simulink model "Appl_VentFault_CtrlModel"  (R2018b)
settings: configuration reference "CodeConfig_1_ms" (kept outside this file)
undefined symbols (not defined in the file): CAL_VentCmdOpenTime, CAL_VentCmdShortTime, FALSE, TRUE
libraries: DareLib x20, simulink x1
settings Model: Creator=Administrator  LastModifiedBy=Administrator
settings ConfigSetRef: SourceLocation=Base Workspace

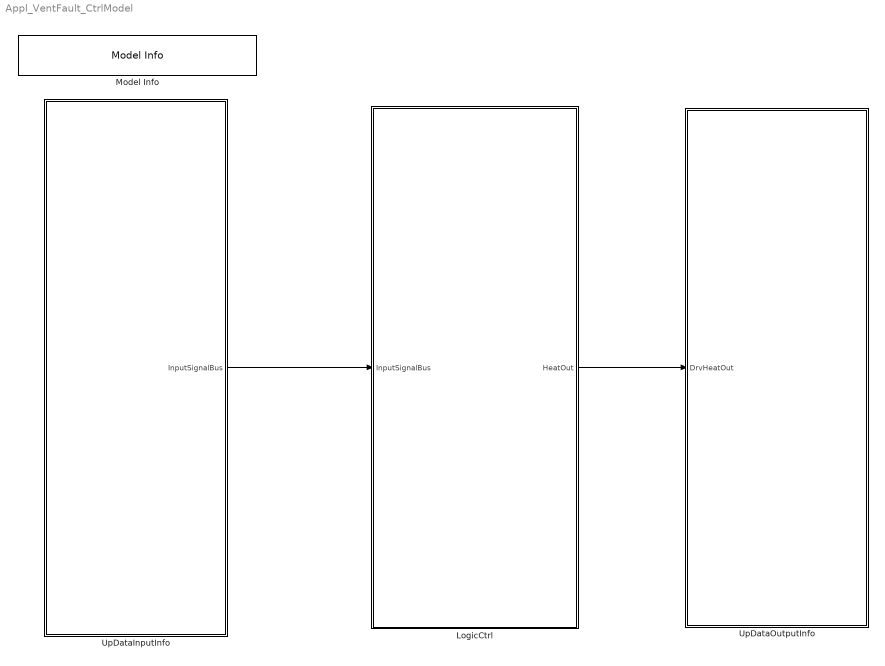
== system Appl_VentFault_CtrlModel ==
  LogicCtrl : Subsystem  Priority=2  TreatAsAtomicUnit=on
      settings: RTWSystemCode=Nonreusable function  RTWFcnNameOpts=Use subsystem name
  Model Info : simulink/Model-Wide Utilities/Model Info  Frame=on  DisplayStringWithTags=Version：%<ModelVersion>  HorizontalTextAlignment=Center  LeftAlignmentValue=0.5
  UpDataInputInfo : Subsystem  Priority=1  TreatAsAtomicUnit=on
      settings: RTWSystemCode=Nonreusable function  RTWFcnNameOpts=Use subsystem name
  UpDataOutputInfo : Subsystem  Priority=3  TreatAsAtomicUnit=on
      settings: RTWSystemCode=Nonreusable function  RTWFcnNameOpts=Use subsystem name
  wires:
  LogicCtrl/1(HeatOut) -> UpDataOutputInfo/1(DrvHeatOut)
  UpDataInputInfo/1(InputSignalBus) -> LogicCtrl/1(InputSignalBus)

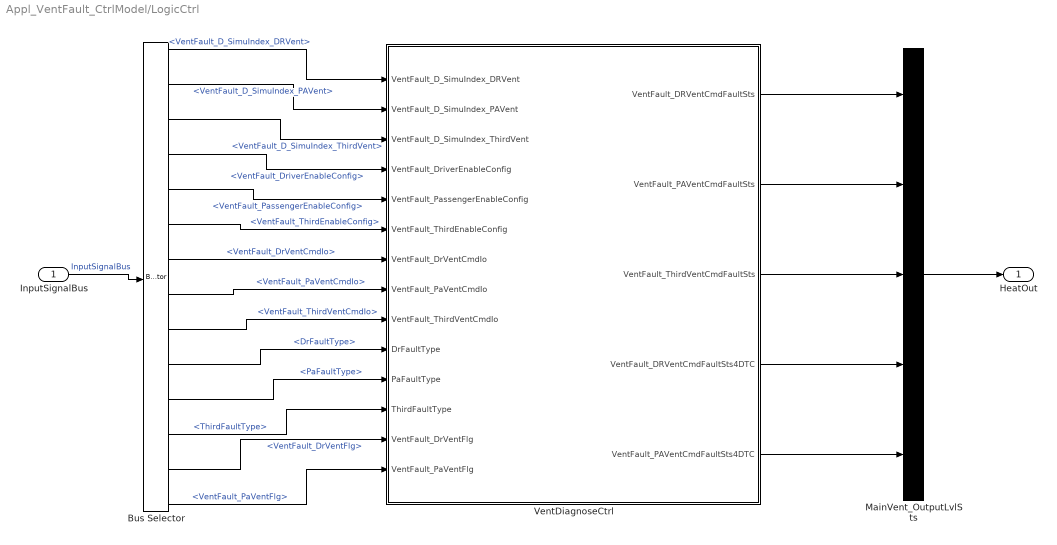
== system Appl_VentFault_CtrlModel/LogicCtrl ==
  InputSignalBus : Inport
  Bus Selector : BusSelector  OutputSignals=Rte_SignalBUs.VentFault_D_SimuIndex_DRVent,Rte_SignalBUs.VentFault_D_SimuIndex_PAVent,Rte_SignalBUs.VentFault_D_SimuIndex_ThirdVent,Rte_SignalBUs.VentFault_DriverEnableConfig,Rte_SignalBUs.VentFault_PassengerEnableConfig,Rte_SignalBUs.VentFault_ThirdEnableConfig,Rte_SignalBUs.VentFault_DrVentCmdIo,Rte_SignalBUs.VentFault_PaVentCmdIo,Rte_SignalBUs.VentFault_ThirdVentCmdIo,DrFaultType,PaFaultType,ThirdFaultType,Rte_SignalBUs.VentFault_DrVentFlg,Rte_SignalBUs.VentFault_PaVentFlg
  MainVent_OutputLvlSts : BusCreator  Inputs=5
  VentDiagnoseCtrl : Subsystem  Description=通风诊断逻辑处理
      settings: AttributesFormatString=%<Description>
  HeatOut : Outport
  wires:
  InputSignalBus/1 -> Bus Selector/1  "InputSignalBus"
  MainVent_OutputLvlSts/1 -> HeatOut/1
  Bus Selector/9 -> VentDiagnoseCtrl/9(VentFault_ThirdVentCmdIo)  "<VentFault_ThirdVentCmdIo>"
  Bus Selector/8 -> VentDiagnoseCtrl/8(VentFault_PaVentCmdIo)  "<VentFault_PaVentCmdIo>"
  Bus Selector/7 -> VentDiagnoseCtrl/7(VentFault_DrVentCmdIo)  "<VentFault_DrVentCmdIo>"
  Bus Selector/6 -> VentDiagnoseCtrl/6(VentFault_ThirdEnableConfig)  "<VentFault_ThirdEnableConfig>"
  Bus Selector/5 -> VentDiagnoseCtrl/5(VentFault_PassengerEnableConfig)  "<VentFault_PassengerEnableConfig>"
  Bus Selector/4 -> VentDiagnoseCtrl/4(VentFault_DriverEnableConfig)  "<VentFault_DriverEnableConfig>"
  Bus Selector/3 -> VentDiagnoseCtrl/3(VentFault_D_SimuIndex_ThirdVent)  "<VentFault_D_SimuIndex_ThirdVent>"
  Bus Selector/2 -> VentDiagnoseCtrl/2(VentFault_D_SimuIndex_PAVent)  "<VentFault_D_SimuIndex_PAVent>"
  Bus Selector/1 -> VentDiagnoseCtrl/1(VentFault_D_SimuIndex_DRVent)  "<VentFault_D_SimuIndex_DRVent>"
  VentDiagnoseCtrl/3(VentFault_ThirdVentCmdFaultSts) -> MainVent_OutputLvlSts/3
  VentDiagnoseCtrl/2(VentFault_PAVentCmdFaultSts) -> MainVent_OutputLvlSts/2
  VentDiagnoseCtrl/1(VentFault_DRVentCmdFaultSts) -> MainVent_OutputLvlSts/1
  VentDiagnoseCtrl/4(VentFault_DRVentCmdFaultSts4DTC) -> MainVent_OutputLvlSts/4
  VentDiagnoseCtrl/5(VentFault_PAVentCmdFaultSts4DTC) -> MainVent_OutputLvlSts/5
  Bus Selector/10 -> VentDiagnoseCtrl/10(DrFaultType)  "<DrFaultType>"
  Bus Selector/11 -> VentDiagnoseCtrl/11(PaFaultType)  "<PaFaultType>"
  Bus Selector/12 -> VentDiagnoseCtrl/12(ThirdFaultType)  "<ThirdFaultType>"
  Bus Selector/13 -> VentDiagnoseCtrl/13(VentFault_DrVentFlg)  "<VentFault_DrVentFlg>"
  Bus Selector/14 -> VentDiagnoseCtrl/14(VentFault_PaVentFlg)  "<VentFault_PaVentFlg>"

== system Appl_VentFault_CtrlModel/UpDataInputInfo ==
  InputSignalProcess : Subsystem  Description=数据处理
      settings: AttributesFormatString=%<Description>  RTWSystemCode=Nonreusable function  RTWFcnNameOpts=Use subsystem name
  RTE : Subsystem  Description=接口自动生成  TreatAsAtomicUnit=on
      settings: AttributesFormatString=%<Description>  RTWSystemCode=Nonreusable function  RTWFcnNameOpts=Use subsystem name
  InputSignalBus : Outport
  wires:
  RTE/1(RTE_Signal) -> InputSignalProcess/1(Rte_SignalBUs)
  InputSignalProcess/1(InputSignalBus) -> InputSignalBus/1

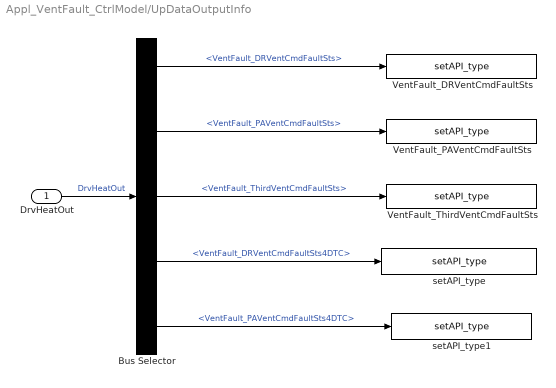
== system Appl_VentFault_CtrlModel/UpDataOutputInfo ==
  DrvHeatOut : Inport
  Bus Selector : BusSelector  OutputSignals=VentFault_DRVentCmdFaultSts,VentFault_PAVentCmdFaultSts,VentFault_ThirdVentCmdFaultSts,VentFault_DRVentCmdFaultSts4DTC,VentFault_PAVentCmdFaultSts4DTC
  VentFault_DRVentCmdFaultSts : DareLib/Dare/setAPI_type  g_funcname=Rte_SetVfb_DrVentCmdFaultSts  g_param=""  g_type=uint8  g_enum=enVentCmdFault  g_size=-1
      settings: AttributesFormatString=%<g_funcname>  SourceProductName=Dare Library
  VentFault_PAVentCmdFaultSts : DareLib/Dare/setAPI_type  g_funcname=Rte_SetVfb_PaVentCmdFaultSts  g_param=""  g_type=uint8  g_enum=enVentCmdFault  g_size=-1
      settings: AttributesFormatString=%<g_funcname>  SourceProductName=Dare Library
  VentFault_ThirdVentCmdFaultSts : DareLib/Dare/setAPI_type  g_funcname=Rte_SetVfb_ThirdVentCmdFaultSts  g_param=""  g_type=uint8  g_enum=enVentCmdFault  g_size=-1
      settings: AttributesFormatString=%<g_funcname>  SourceProductName=Dare Library
  setAPI_type : DareLib/Dare/setAPI_type  g_funcname=Rte_SetVfb_DrVentCmdFaultSts4DTC  g_param=""  g_type=uint8  g_size=-1
      settings: AttributesFormatString=%<g_funcname>  SourceProductName=Dare Library
  setAPI_type1 : DareLib/Dare/setAPI_type  g_funcname=Rte_SetVfb_PaVentCmdFaultSts4DTC  g_param=""  g_type=uint8  g_size=-1
      settings: AttributesFormatString=%<g_funcname>  SourceProductName=Dare Library
  wires:
  DrvHeatOut/1 -> Bus Selector/1  "DrvHeatOut"
  Bus Selector/2 -> VentFault_PAVentCmdFaultSts/1  "<VentFault_PAVentCmdFaultSts>"
  Bus Selector/1 -> VentFault_DRVentCmdFaultSts/1  "<VentFault_DRVentCmdFaultSts>"
  Bus Selector/3 -> VentFault_ThirdVentCmdFaultSts/1  "<VentFault_ThirdVentCmdFaultSts>"
  Bus Selector/4 -> setAPI_type/1  "<VentFault_DRVentCmdFaultSts4DTC>"
  Bus Selector/5 -> setAPI_type1/1  "<VentFault_PAVentCmdFaultSts4DTC>"

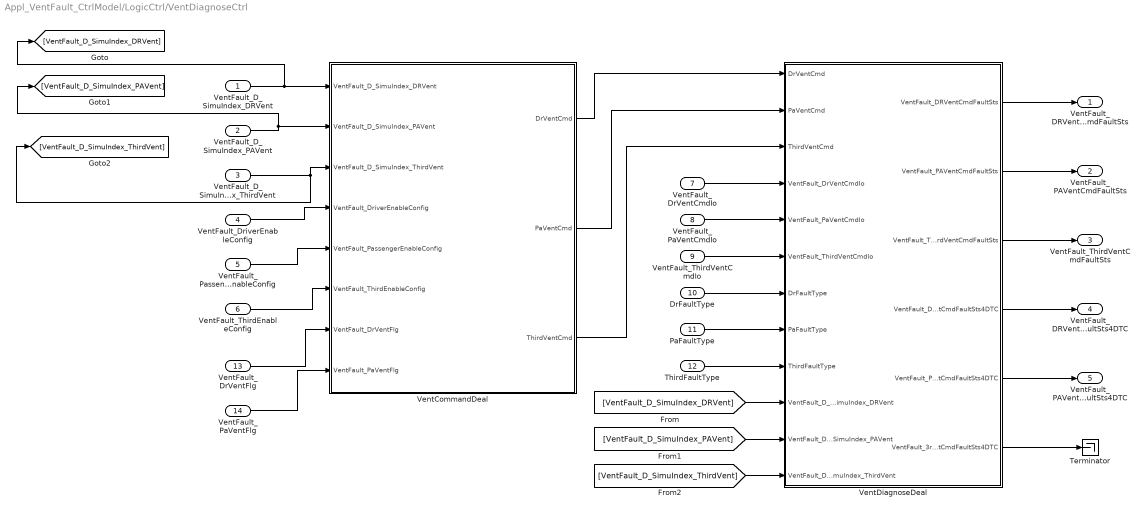
== system Appl_VentFault_CtrlModel/LogicCtrl/VentDiagnoseCtrl ==
  VentFault_D_SimuIndex_DRVent : Inport
  VentFault_D_SimuIndex_PAVent : Inport  Port=2
  VentFault_D_SimuIndex_ThirdVent : Inport  Port=3
  VentFault_DriverEnableConfig : Inport  Port=4
  VentFault_PassengerEnableConfig : Inport  Port=5
  VentFault_ThirdEnableConfig : Inport  Port=6
  VentFault_DrVentCmdIo : Inport  Port=7
  VentFault_PaVentCmdIo : Inport  Port=8
  VentFault_ThirdVentCmdIo : Inport  Port=9
  DrFaultType : Inport  Port=10
  PaFaultType : Inport  Port=11
  ThirdFaultType : Inport  Port=12
  VentFault_DrVentFlg : Inport  Port=13
  VentFault_PaVentFlg : Inport  Port=14
  Terminator : Terminator
  VentCommandDeal : Stateflow chart  TreatAsAtomicUnit=on
  VentDiagnoseDeal : Stateflow chart  TreatAsAtomicUnit=on
  VentFault_DRVentCmdFaultSts : Outport
  VentFault_PAVentCmdFaultSts : Outport  Port=2
  VentFault_ThirdVentCmdFaultSts : Outport  Port=3
  VentFault_DRVentCmdFaultSts4DTC : Outport  Port=4
  VentFault_PAVentCmdFaultSts4DTC : Outport  Port=5
  wires:
  VentDiagnoseDeal/3(VentFault_ThirdVentCmdFaultSts) -> VentFault_ThirdVentCmdFaultSts/1
  VentDiagnoseDeal/2(VentFault_PAVentCmdFaultSts) -> VentFault_PAVentCmdFaultSts/1
  VentDiagnoseDeal/1(VentFault_DRVentCmdFaultSts) -> VentFault_DRVentCmdFaultSts/1
  VentFault_D_SimuIndex_DRVent/1 -> [VentFault_D_SimuIndex_DRVent], VentCommandDeal/1(VentFault_D_SimuIndex_DRVent)
  VentFault_D_SimuIndex_PAVent/1 -> [VentFault_D_SimuIndex_PAVent], VentCommandDeal/2(VentFault_D_SimuIndex_PAVent)
  VentFault_D_SimuIndex_ThirdVent/1 -> [VentFault_D_SimuIndex_ThirdVent], VentCommandDeal/3(VentFault_D_SimuIndex_ThirdVent)
  VentCommandDeal/1(DrVentCmd) -> VentDiagnoseDeal/1(DrVentCmd)
  VentCommandDeal/2(PaVentCmd) -> VentDiagnoseDeal/2(PaVentCmd)
  VentCommandDeal/3(ThirdVentCmd) -> VentDiagnoseDeal/3(ThirdVentCmd)
  VentFault_DriverEnableConfig/1 -> VentCommandDeal/4(VentFault_DriverEnableConfig)
  VentFault_PassengerEnableConfig/1 -> VentCommandDeal/5(VentFault_PassengerEnableConfig)
  VentFault_ThirdEnableConfig/1 -> VentCommandDeal/6(VentFault_ThirdEnableConfig)
  VentFault_DrVentCmdIo/1 -> VentDiagnoseDeal/4(VentFault_DrVentCmdIo)
  VentFault_PaVentCmdIo/1 -> VentDiagnoseDeal/5(VentFault_PaVentCmdIo)
  VentFault_ThirdVentCmdIo/1 -> VentDiagnoseDeal/6(VentFault_ThirdVentCmdIo)
  VentDiagnoseDeal/5(VentFault_PAVentCmdFaultSts4DTC) -> VentFault_PAVentCmdFaultSts4DTC/1
  VentDiagnoseDeal/4(VentFault_DRVentCmdFaultSts4DTC) -> VentFault_DRVentCmdFaultSts4DTC/1
  DrFaultType/1 -> VentDiagnoseDeal/7(DrFaultType)
  PaFaultType/1 -> VentDiagnoseDeal/8(PaFaultType)
  ThirdFaultType/1 -> VentDiagnoseDeal/9(ThirdFaultType)
  VentDiagnoseDeal/6(VentFault_3rdVentCmdFaultSts4DTC) -> Terminator/1
  [VentFault_D_SimuIndex_DRVent] -> VentDiagnoseDeal/10(VentFault_D_SimuIndex_DRVent)
  [VentFault_D_SimuIndex_PAVent] -> VentDiagnoseDeal/11(VentFault_D_SimuIndex_PAVent)
  [VentFault_D_SimuIndex_ThirdVent] -> VentDiagnoseDeal/12(VentFault_D_SimuIndex_ThirdVent)
  VentFault_PaVentFlg/1 -> VentCommandDeal/8(VentFault_PaVentFlg)
  VentFault_DrVentFlg/1 -> VentCommandDeal/7(VentFault_DrVentFlg)

== system Appl_VentFault_CtrlModel/UpDataInputInfo/InputSignalProcess ==
  Rte_SignalBUs : Inport
  Bus Creator : BusCreator  Inputs=4
  Bus Selector : BusSelector  OutputSignals=VentFault_DrPWMShortGND,VentFault_DrPWMShortPWR,VentFault_PaPWMShortGND,VentFault_PaPWMShortPWR
  PWM_Process : Subsystem  Description=PWM诊断DTC处理（确认当前PWM有哪个DTC）
      settings: AttributesFormatString=%<Description>
  InputSignalBus : Outport
  wires:
  Bus Creator/1 -> InputSignalBus/1
  Rte_SignalBUs/1 -> Bus Selector/1, Bus Creator/1  "Rte_SignalBUs"
  Bus Selector/1 -> PWM_Process/1(VentFault_DrPWMShortGND)  "<VentFault_DrPWMShortGND>"
  Bus Selector/2 -> PWM_Process/2(VentFault_DrPWMShortPWR)  "<VentFault_DrPWMShortPWR>"
  Bus Selector/3 -> PWM_Process/3(VentFault_PaPWMShortGND)  "<VentFault_PaPWMShortGND>"
  Bus Selector/4 -> PWM_Process/4(VentFault_PaPWMShortPWR)  "<VentFault_PaPWMShortPWR>"
  PWM_Process/1(DrFaultType) -> Bus Creator/2
  PWM_Process/2(PaFaultType) -> Bus Creator/3
  PWM_Process/3(ThirdFaultType) -> Bus Creator/4

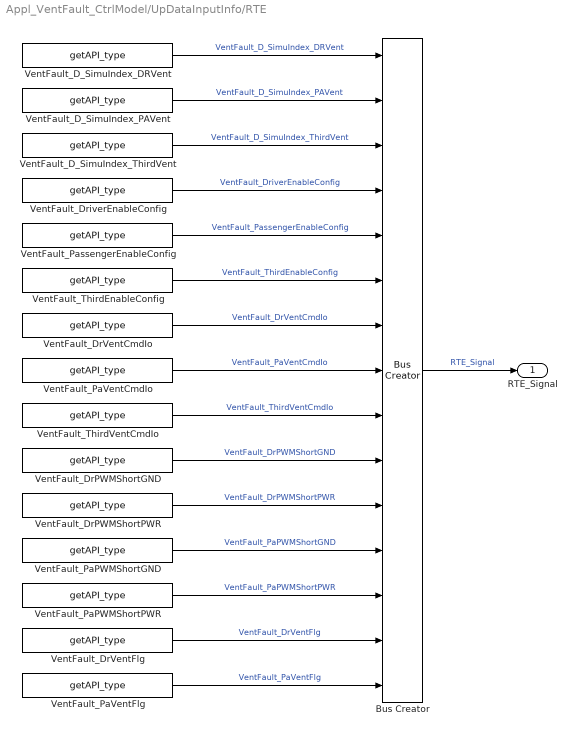
== system Appl_VentFault_CtrlModel/UpDataInputInfo/RTE ==
  Bus Creator : BusCreator  Inputs=15
  VentFault_D_SimuIndex_DRVent : DareLib/Dare/getAPI_type  g_funcname=Rte_GetVfb_DrVent  g_param=""  g_type=uint8  g_enum=enVentLvlSts  g_size=-1
      settings: AttributesFormatString=%<g_funcname>  SourceProductName=Dare Library
  VentFault_D_SimuIndex_PAVent : DareLib/Dare/getAPI_type  g_funcname=Rte_GetVfb_PaVent  g_param=""  g_type=uint8  g_enum=enVentLvlSts  g_size=-1
      settings: AttributesFormatString=%<g_funcname>  SourceProductName=Dare Library
  VentFault_D_SimuIndex_ThirdVent : DareLib/Dare/getAPI_type  g_funcname=Rte_GetVfb_ThirdVent  g_param=""  g_type=uint8  g_enum=enVentLvlSts  g_size=-1
      settings: AttributesFormatString=%<g_funcname>  SourceProductName=Dare Library
  VentFault_DrPWMShortGND : DareLib/Dare/getAPI_type  g_funcname=Diag_ReadDtcTestFailFlag  g_param=D_DTC_DrVentPWMGS  g_type=uint8  g_size=-1
      settings: AttributesFormatString=%<g_funcname>  SourceProductName=Dare Library
  VentFault_DrPWMShortPWR : DareLib/Dare/getAPI_type  g_funcname=Diag_ReadDtcTestFailFlag  g_param=D_DTC_DrVentPWMPS  g_type=uint8  g_size=-1
      settings: AttributesFormatString=%<g_funcname>  SourceProductName=Dare Library
  VentFault_DrVentCmdIo : DareLib/Dare/getAPI_type  g_funcname=Ecual_GetDigitalSwStatus  g_param=EN_DRVenFeedback  g_type=uint8  g_size=-1
      settings: AttributesFormatString=%<g_funcname>  SourceProductName=Dare Library
  VentFault_DrVentFlg : DareLib/Dare/getAPI_type  g_funcname=Rte_GetVfb_DrVentEnable  g_param=""  g_type=uint8  g_size=-1
      settings: AttributesFormatString=%<g_funcname>  SourceProductName=Dare Library
  VentFault_DriverEnableConfig : DareLib/Dare/getAPI_type  g_funcname=Rte_GetVfb_DrVentEnable  g_param=""  g_type=uint8  g_size=-1
      settings: AttributesFormatString=%<g_funcname>  SourceProductName=Dare Library
  VentFault_PaPWMShortGND : DareLib/Dare/getAPI_type  g_funcname=Diag_ReadDtcTestFailFlag  g_param=D_DTC_PaVentPWMGS  g_type=uint8  g_size=-1
      settings: AttributesFormatString=%<g_funcname>  SourceProductName=Dare Library
  VentFault_PaPWMShortPWR : DareLib/Dare/getAPI_type  g_funcname=Diag_ReadDtcTestFailFlag  g_param=D_DTC_PaVentPWMPS  g_type=uint8  g_size=-1
      settings: AttributesFormatString=%<g_funcname>  SourceProductName=Dare Library
  VentFault_PaVentCmdIo : DareLib/Dare/getAPI_type  g_funcname=Ecual_GetDigitalSwStatus  g_param=EN_PaVenFeedback  g_type=uint8  g_size=-1
      settings: AttributesFormatString=%<g_funcname>  SourceProductName=Dare Library
  VentFault_PaVentFlg : DareLib/Dare/getAPI_type  g_funcname=Rte_GetVfb_SecondVentEnable  g_param=""  g_type=uint8  g_size=-1
      settings: AttributesFormatString=%<g_funcname>  SourceProductName=Dare Library
  VentFault_PassengerEnableConfig : DareLib/Dare/getAPI_type  g_funcname=Rte_GetVfb_SecondVentEnable  g_param=""  g_type=uint8  g_size=-1
      settings: AttributesFormatString=%<g_funcname>  SourceProductName=Dare Library
  VentFault_ThirdEnableConfig : DareLib/Dare/getAPI_type  g_funcname=Rte_GetVfb_ThirdVentEnable  g_param=""  g_type=uint8  g_size=-1
      settings: AttributesFormatString=%<g_funcname>  SourceProductName=Dare Library
  VentFault_ThirdVentCmdIo : DareLib/Dare/getAPI_type  g_funcname=Vfb_Reserved_0  g_param=""  g_type=uint8  g_size=-1
      settings: AttributesFormatString=%<g_funcname>  SourceProductName=Dare Library
  RTE_Signal : Outport
  wires:
  Bus Creator/1 -> RTE_Signal/1  "RTE_Signal"
  VentFault_D_SimuIndex_DRVent/1 -> Bus Creator/1  "VentFault_D_SimuIndex_DRVent"
  VentFault_D_SimuIndex_PAVent/1 -> Bus Creator/2  "VentFault_D_SimuIndex_PAVent"
  VentFault_D_SimuIndex_ThirdVent/1 -> Bus Creator/3  "VentFault_D_SimuIndex_ThirdVent"
  VentFault_DriverEnableConfig/1 -> Bus Creator/4  "VentFault_DriverEnableConfig"
  VentFault_PassengerEnableConfig/1 -> Bus Creator/5  "VentFault_PassengerEnableConfig"
  VentFault_ThirdEnableConfig/1 -> Bus Creator/6  "VentFault_ThirdEnableConfig"
  VentFault_DrVentCmdIo/1 -> Bus Creator/7  "VentFault_DrVentCmdIo"
  VentFault_PaVentCmdIo/1 -> Bus Creator/8  "VentFault_PaVentCmdIo"
  VentFault_ThirdVentCmdIo/1 -> Bus Creator/9  "VentFault_ThirdVentCmdIo"
  VentFault_DrPWMShortGND/1 -> Bus Creator/10  "VentFault_DrPWMShortGND"
  VentFault_DrPWMShortPWR/1 -> Bus Creator/11  "VentFault_DrPWMShortPWR"
  VentFault_PaPWMShortGND/1 -> Bus Creator/12  "VentFault_PaPWMShortGND"
  VentFault_PaPWMShortPWR/1 -> Bus Creator/13  "VentFault_PaPWMShortPWR"
  VentFault_DrVentFlg/1 -> Bus Creator/14  "VentFault_DrVentFlg"
  VentFault_PaVentFlg/1 -> Bus Creator/15  "VentFault_PaVentFlg"

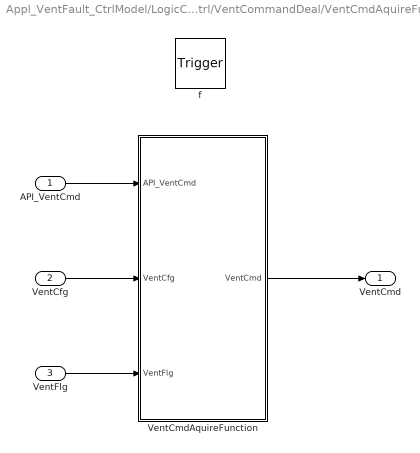
== system Appl_VentFault_CtrlModel/LogicCtrl/VentDiagnoseCtrl/VentCommandDeal/VentCmdAquireFunction ==
  API_VentCmd : Inport
  VentCfg : Inport  Port=2
  VentFlg : Inport  Port=3
  f : TriggerPort  TriggerType=function-call  VariantControl=(inherit)
      settings: CopyFcn=Stateflow.SLINSF.SimulinkMan.removeBlockPreDeleteFcn  PreDeleteFcn=Stateflow.SLINSF.SimulinkMan.unsafePredeleteFcn
  VentCmdAquireFunction : Stateflow chart  TreatAsAtomicUnit=on
  VentCmd : Outport
  wires:
  VentCfg/1 -> VentCmdAquireFunction/2(VentCfg)
  API_VentCmd/1 -> VentCmdAquireFunction/1(API_VentCmd)
  VentCmdAquireFunction/1(VentCmd) -> VentCmd/1
  VentFlg/1 -> VentCmdAquireFunction/3(VentFlg)

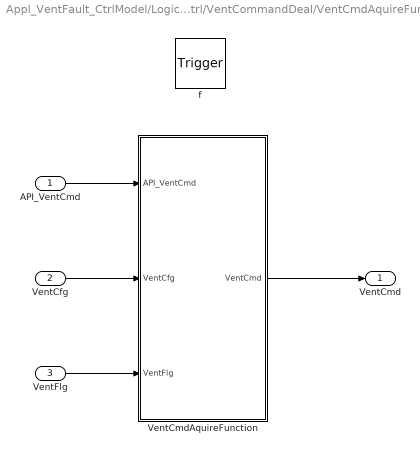
== system Appl_VentFault_CtrlModel/LogicCtrl/VentDiagnoseCtrl/VentCommandDeal/VentCmdAquireFunction1 ==
  API_VentCmd : Inport
  VentCfg : Inport  Port=2
  VentFlg : Inport  Port=3
  f : TriggerPort  TriggerType=function-call  VariantControl=(inherit)
      settings: CopyFcn=Stateflow.SLINSF.SimulinkMan.removeBlockPreDeleteFcn  PreDeleteFcn=Stateflow.SLINSF.SimulinkMan.unsafePredeleteFcn
  VentCmdAquireFunction : Stateflow chart  TreatAsAtomicUnit=on
  VentCmd : Outport
  wires:
  VentCfg/1 -> VentCmdAquireFunction/2(VentCfg)
  API_VentCmd/1 -> VentCmdAquireFunction/1(API_VentCmd)
  VentCmdAquireFunction/1(VentCmd) -> VentCmd/1
  VentFlg/1 -> VentCmdAquireFunction/3(VentFlg)

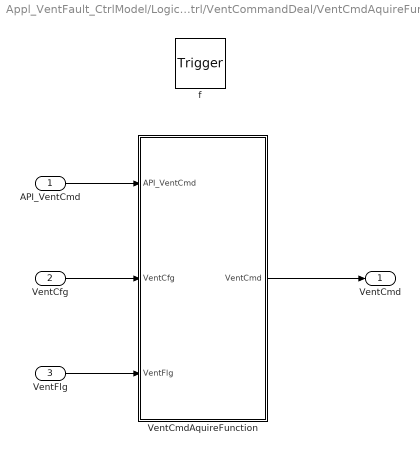
== system Appl_VentFault_CtrlModel/LogicCtrl/VentDiagnoseCtrl/VentCommandDeal/VentCmdAquireFunction2 ==
  API_VentCmd : Inport
  VentCfg : Inport  Port=2
  VentFlg : Inport  Port=3
  f : TriggerPort  TriggerType=function-call  VariantControl=(inherit)
      settings: CopyFcn=Stateflow.SLINSF.SimulinkMan.removeBlockPreDeleteFcn  PreDeleteFcn=Stateflow.SLINSF.SimulinkMan.unsafePredeleteFcn
  VentCmdAquireFunction : Stateflow chart  TreatAsAtomicUnit=on
  VentCmd : Outport
  wires:
  VentCfg/1 -> VentCmdAquireFunction/2(VentCfg)
  API_VentCmd/1 -> VentCmdAquireFunction/1(API_VentCmd)
  VentCmdAquireFunction/1(VentCmd) -> VentCmd/1
  VentFlg/1 -> VentCmdAquireFunction/3(VentFlg)

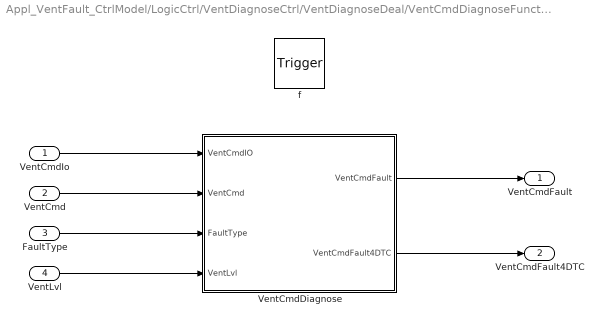
== system Appl_VentFault_CtrlModel/LogicCtrl/VentDiagnoseCtrl/VentDiagnoseDeal/VentCmdDiagnoseFunction ==
  VentCmdIo : Inport
  VentCmd : Inport  Port=2
  FaultType : Inport  Port=3
  VentLvl : Inport  Port=4
  f : TriggerPort  TriggerType=function-call  VariantControl=(inherit)
      settings: CopyFcn=Stateflow.SLINSF.SimulinkMan.removeBlockPreDeleteFcn  PreDeleteFcn=Stateflow.SLINSF.SimulinkMan.unsafePredeleteFcn
  VentCmdDiagnose : Stateflow chart  TreatAsAtomicUnit=on
  VentCmdFault : Outport
  VentCmdFault4DTC : Outport  Port=2
  wires:
  VentCmdIo/1 -> VentCmdDiagnose/1(VentCmdIO)
  VentCmdDiagnose/1(VentCmdFault) -> VentCmdFault/1
  VentCmd/1 -> VentCmdDiagnose/2(VentCmd)
  VentCmdDiagnose/2(VentCmdFault4DTC) -> VentCmdFault4DTC/1
  FaultType/1 -> VentCmdDiagnose/3(FaultType)
  VentLvl/1 -> VentCmdDiagnose/4(VentLvl)

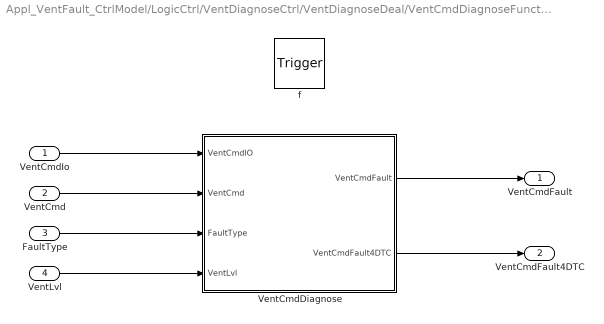
== system Appl_VentFault_CtrlModel/LogicCtrl/VentDiagnoseCtrl/VentDiagnoseDeal/VentCmdDiagnoseFunction1 ==
  VentCmdIo : Inport
  VentCmd : Inport  Port=2
  FaultType : Inport  Port=3
  VentLvl : Inport  Port=4
  f : TriggerPort  TriggerType=function-call  VariantControl=(inherit)
      settings: CopyFcn=Stateflow.SLINSF.SimulinkMan.removeBlockPreDeleteFcn  PreDeleteFcn=Stateflow.SLINSF.SimulinkMan.unsafePredeleteFcn
  VentCmdDiagnose : Stateflow chart  TreatAsAtomicUnit=on
  VentCmdFault : Outport
  VentCmdFault4DTC : Outport  Port=2
  wires:
  VentCmdIo/1 -> VentCmdDiagnose/1(VentCmdIO)
  VentCmdDiagnose/1(VentCmdFault) -> VentCmdFault/1
  VentCmd/1 -> VentCmdDiagnose/2(VentCmd)
  VentCmdDiagnose/2(VentCmdFault4DTC) -> VentCmdFault4DTC/1
  FaultType/1 -> VentCmdDiagnose/3(FaultType)
  VentLvl/1 -> VentCmdDiagnose/4(VentLvl)

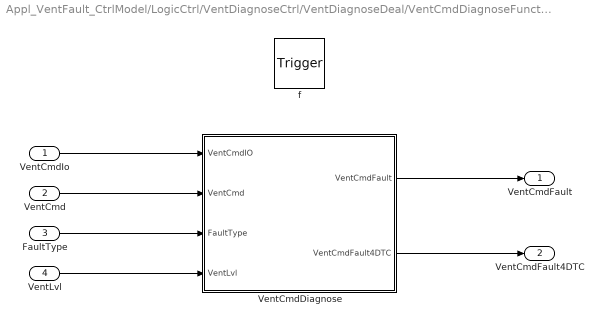
== system Appl_VentFault_CtrlModel/LogicCtrl/VentDiagnoseCtrl/VentDiagnoseDeal/VentCmdDiagnoseFunction2 ==
  VentCmdIo : Inport
  VentCmd : Inport  Port=2
  FaultType : Inport  Port=3
  VentLvl : Inport  Port=4
  f : TriggerPort  TriggerType=function-call  VariantControl=(inherit)
      settings: CopyFcn=Stateflow.SLINSF.SimulinkMan.removeBlockPreDeleteFcn  PreDeleteFcn=Stateflow.SLINSF.SimulinkMan.unsafePredeleteFcn
  VentCmdDiagnose : Stateflow chart  TreatAsAtomicUnit=on
  VentCmdFault : Outport
  VentCmdFault4DTC : Outport  Port=2
  wires:
  VentCmdIo/1 -> VentCmdDiagnose/1(VentCmdIO)
  VentCmdDiagnose/1(VentCmdFault) -> VentCmdFault/1
  VentCmd/1 -> VentCmdDiagnose/2(VentCmd)
  VentCmdDiagnose/2(VentCmdFault4DTC) -> VentCmdFault4DTC/1
  FaultType/1 -> VentCmdDiagnose/3(FaultType)
  VentLvl/1 -> VentCmdDiagnose/4(VentLvl)

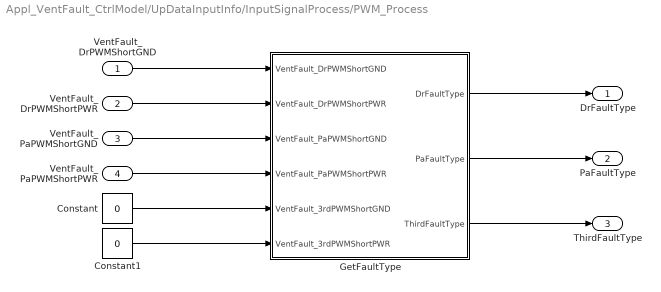
== system Appl_VentFault_CtrlModel/UpDataInputInfo/InputSignalProcess/PWM_Process ==
  VentFault_DrPWMShortGND : Inport
  VentFault_DrPWMShortPWR : Inport  Port=2
  VentFault_PaPWMShortGND : Inport  Port=3
  VentFault_PaPWMShortPWR : Inport  Port=4
  Constant : Constant  Value=0
  Constant1 : Constant  Value=0
  GetFaultType : Stateflow chart  TreatAsAtomicUnit=on
  DrFaultType : Outport
  PaFaultType : Outport  Port=2
  ThirdFaultType : Outport  Port=3
  wires:
  GetFaultType/1(DrFaultType) -> DrFaultType/1
  VentFault_DrPWMShortGND/1 -> GetFaultType/1(VentFault_DrPWMShortGND)
  VentFault_DrPWMShortPWR/1 -> GetFaultType/2(VentFault_DrPWMShortPWR)
  VentFault_PaPWMShortGND/1 -> GetFaultType/3(VentFault_PaPWMShortGND)
  VentFault_PaPWMShortPWR/1 -> GetFaultType/4(VentFault_PaPWMShortPWR)
  GetFaultType/2(PaFaultType) -> PaFaultType/1
  GetFaultType/3(ThirdFaultType) -> ThirdFaultType/1
  Constant/1 -> GetFaultType/5(VentFault_3rdPWMShortGND)
  Constant1/1 -> GetFaultType/6(VentFault_3rdPWMShortPWR)

== system Appl_VentFault_CtrlModel/UpDataInputInfo/InputSignalProcess/PWM_Process/GetFaultType/getFaultType ==
  ShortGND : Inport
  ShortPWR : Inport  Port=2
  f : TriggerPort  TriggerType=function-call  VariantControl=(inherit)
      settings: CopyFcn=Stateflow.SLINSF.SimulinkMan.removeBlockPreDeleteFcn  PreDeleteFcn=Stateflow.SLINSF.SimulinkMan.unsafePredeleteFcn
  Chart : Stateflow chart  TreatAsAtomicUnit=on
  FaultType : Outport
  wires:
  Chart/1(VentPWMFault) -> FaultType/1
  ShortGND/1 -> Chart/1(VentPWMGS)
  ShortPWR/1 -> Chart/2(VentPWMSP)

== stateflow chart Appl_VentFault_CtrlModel/LogicCtrl/VentDiagnoseCtrl/VentCommandDeal ==
  state VentCmd = VentCmdAquireFunction(API_VentCmd,VentCfg,VentFlg) [function]
  state VentCmd = VentCmdAquireFunction1(API_VentCmd,VentCfg,VentFlg) [function]
  state VentCmd = VentCmdAquireFunction2(API_VentCmd,VentCfg,VentFlg) [function]
  state DriverVentCommandDeal [parallel]
    du:
    DrVentCmd = VentCmdAquireFunction(VentFault_D_SimuIndex_DRVent,VentFault_DriverEnableConfig,VentFault_DrVentFlg);
    settings: executionOrder=1
  state PassengerVentCommandDeal [parallel]
    du:
    PaVentCmd = VentCmdAquireFunction1(VentFault_D_SimuIndex_PAVent,VentFault_PassengerEnableConfig,VentFault_PaVentFlg);
    settings: executionOrder=2
  state ThirdVentCommandDeal [parallel]
    du:
    ThirdVentCmd = VentCmdAquireFunction2(VentFault_D_SimuIndex_ThirdVent,VentFault_ThirdEnableConfig,TRUE);
    settings: executionOrder=3
  data: API_VentCmd function_input; VentCfg function_input; VentCmd function_output; VentFlg function_input; API_VentCmd function_input; VentCfg function_input; VentCmd function_output; VentFlg function_input; API_VentCmd function_input; VentCfg function_input; VentCmd function_output; VentFlg function_input; VentFault_D_SimuIndex_DRVent input; VentFault_D_SimuIndex_PAVent input; VentFault_D_SimuIndex_ThirdVent input; VentFault_DriverEnableConfig input; VentFault_PassengerEnableConfig input; VentFault_ThirdEnableConfig input; DrVentCmd output uint8; PaVentCmd output uint8; ThirdVentCmd output uint8; VentFault_DrVentFlg input; VentFault_PaVentFlg input; TRUE parameter

== stateflow chart Appl_VentFault_CtrlModel/LogicCtrl/VentDiagnoseCtrl/VentCommandDeal/VentCmdAquireFunction/VentCmdAquireFunction ==
  state HeatCmdInvalid
    en:
    VentCmd = FALSE;
  state HeatCmdValid
    en:
    VentCmd = TRUE;
  (default) -> HeatCmdInvalid
  HeatCmdInvalid -> HeatCmdValid : /* 指令有效 */
      | [enVentLvlSts.EN_VENT_LVL_OFF != API_VentCmd ...
      | && TRUE == VentCfg && TRUE == VentFlg]
  HeatCmdValid -> HeatCmdInvalid : /* 指令无效 */
      | [enVentLvlSts.EN_VENT_LVL_OFF == API_VentCmd ...
      | || TRUE != VentCfg || TRUE != VentFlg]
  data: API_VentCmd input Enum: enVentLvlSts; VentCfg input uint8; TRUE parameter; VentCmd output uint8; FALSE parameter; VentFlg input uint8

== stateflow chart Appl_VentFault_CtrlModel/LogicCtrl/VentDiagnoseCtrl/VentDiagnoseDeal ==
  state [VentCmdFault,VentCmdFault4DTC] = VentCmdDiagnoseFunction(VentCmdIo,VentCmd,FaultType,VentLvl) [function]
  state [VentCmdFault,VentCmdFault4DTC] = VentCmdDiagnoseFunction1(VentCmdIo,VentCmd,FaultType,VentLvl) [function]
  state [VentCmdFault,VentCmdFault4DTC] = VentCmdDiagnoseFunction2(VentCmdIo,VentCmd,FaultType,VentLvl) [function]
  state Driver_VentDiagnose [parallel]
    du:
    [VentFault_DRVentCmdFaultSts,VentFault_DRVentCmdFaultSts4DTC] = VentCmdDiagnoseFunction(VentFault_DrVentCmdIo,DrVentCmd,DrFaultType,VentFault_D_SimuIndex_DRVent);
    settings: executionOrder=1
  state Passenger_VentDiagnose [parallel]
    du:
    [VentFault_PAVentCmdFaultSts ,VentFault_PAVentCmdFaultSts4DTC] = VentCmdDiagnoseFunction1(VentFault_PaVentCmdIo,PaVentCmd,PaFaultType,VentFault_D_SimuIndex_PAVent);
    settings: executionOrder=2
  state Third_VentDiagnose [parallel]
    du:
    [VentFault_ThirdVentCmdFaultSts,VentFault_3rdVentCmdFaultSts4DTC] = VentCmdDiagnoseFunction2(VentFault_ThirdVentCmdIo,ThirdVentCmd,ThirdFaultType,VentFault_D_SimuIndex_ThirdVent);
    settings: executionOrder=3
  data: VentCmdIo function_input; VentCmd function_input; VentCmdFault function_output; VentCmdFault4DTC function_output; FaultType function_input; VentLvl function_input; VentCmdIo function_input; VentCmd function_input; VentCmdFault function_output; VentCmdFault4DTC function_output; FaultType function_input; VentLvl function_input; VentCmdIo function_input; VentCmd function_input; VentCmdFault function_output; VentCmdFault4DTC function_output; FaultType function_input; VentLvl function_input; DrVentCmd input; PaVentCmd input; ThirdVentCmd input; VentFault_DrVentCmdIo input; VentFault_PaVentCmdIo input; VentFault_ThirdVentCmdIo input; VentFault_DRVentCmdFaultSts output Enum: enVentCmdFault; VentFault_PAVentCmdFaultSts output Enum: enVentCmdFault; VentFault_ThirdVentCmdFaultSts output Enum: enVentCmdFault; VentFault_DRVentCmdFaultSts4DTC output uint8; VentFault_PAVentCmdFaultSts4DTC output uint8; DrFaultType input; PaFaultType input; ThirdFaultType input; VentFault_3rdVentCmdFaultSts4DTC output uint8; VentFault_D_SimuIndex_DRVent input; VentFault_D_SimuIndex_PAVent input; VentFault_D_SimuIndex_ThirdVent input

== stateflow chart Appl_VentFault_CtrlModel/LogicCtrl/VentDiagnoseCtrl/VentDiagnoseDeal/VentCmdDiagnoseFunction/VentCmdDiagnose ==
  state HeatCmdDiagnosis
    state CmdShortToPower
      ex:
      ShortTimer = 0;
      (default) -> (junction 25)
      CmdShortToPower -> (junction 25) [order 1]
      (junction 25) -> (junction 28) [order 1] : /* 未超时 */
          | [CAL_VentCmdShortTime > ShortTimer]
      (junction 25) -> (junction 30) [order 2] : {/*设置DTC故障标志位，关闭事件报文主驾通风档位*/
          | ShortTimer = CAL_VentCmdShortTime;
          | VentCmdFault = enVentCmdFault.EN_VENT_FAULT_LOAD;
          | VentCmdFault4DTC = enVentCmdFault.EN_VENT_FAULT_LOAD;
          | }
      (junction 28) -> (junction 32) : {ShortTimer++;}
      (junction 32) -> (junction 30)
      (junction 30) -> (junction 35)
    state Default
      en:
      OpenTimer = 0;
      ShortTimer = 0;
      VentCmdFault =  enVentCmdFault.EN_VENT_FAULT_NONE;
      VentCmdFault4DTC =  enVentCmdFault.EN_VENT_FAULT_NONE;
    state CmdOpenLoad
      ex:
      OpenTimer = 0;
      (default) -> (junction 46)
      CmdOpenLoad -> (junction 46) [order 1]
      (junction 46) -> (junction 43) [order 1] : /* 未超时 */
          | [CAL_VentCmdOpenTime > OpenTimer]
      (junction 46) -> (junction 47) [order 2] : {/*设置DTC故障标志位，关闭事件报文主驾通风档位*/
          | OpenTimer = CAL_VentCmdOpenTime;
          | VentCmdFault = enVentCmdFault.EN_VENT_FAULT_OPEN;
          | VentCmdFault4DTC = enVentCmdFault.EN_VENT_FAULT_OPEN;
          | }
      (junction 43) -> (junction 48) : {OpenTimer++;}
      (junction 48) -> (junction 47)
      (junction 47) -> (junction 40)
    (junction 78) -> CmdShortToPower [order 1] : [FaultType ==enVentCmdFault.EN_VENT_FAULT_LOAD]
    Default -> CmdShortToPower [order 1] : /* pwm输出为高 */
        | [TRUE == VentCmdIO]
    CmdShortToPower -> Default [order 1] : /* pwm输出为低 */
        | [FALSE == VentCmdIO]
    (default) -> (junction 78)
    (junction 78) -> Default [order 3]
    (junction 78) -> CmdOpenLoad [order 2] : [FaultType ==enVentCmdFault.EN_VENT_FAULT_OPEN]
    Default -> CmdOpenLoad [order 2] : /* pwm输出为低 且不为 3档*/
        | [FALSE == VentCmdIO ...
        | && VentLvl != enVentLvlSts.EN_VENT_LVL_3]
    CmdOpenLoad -> Default [order 1] : /* pwm输出为高 或为3档*/
        | [TRUE == VentCmdIO ...
        | || VentLvl == enVentLvlSts.EN_VENT_LVL_3]
  state VentCmdClose
    en:
    OpenTimer = 0;
    ShortTimer = 0;
    VentCmdFault = enVentCmdFault.EN_VENT_FAULT_NONE;
    ex:
    VentCmdFault4DTC = FaultType;
  (default) -> VentCmdClose
  VentCmdClose -> HeatCmdDiagnosis : /* 通风CMD */
      | [TRUE == VentCmd]
  HeatCmdDiagnosis -> VentCmdClose : /* 无通风CMD */
      | [TRUE != VentCmd]
  data: VentCmdIO input Enum: enHeatIoSts; VentCmd input uint8; VentCmdFault output Enum: enVentCmdFault; ShortTimer local uint16; OpenTimer local uint16; CAL_VentCmdShortTime parameter; CAL_VentCmdOpenTime parameter; TRUE parameter; FALSE parameter; VentCmdFault4DTC output uint8; FaultType input Enum: enVentCmdFault; VentLvl input Enum: enVentLvlSts

== stateflow chart Appl_VentFault_CtrlModel/LogicCtrl/VentDiagnoseCtrl/VentCommandDeal/VentCmdAquireFunction1/VentCmdAquireFunction ==
  state HeatCmdInvalid
    en:
    VentCmd = FALSE;
  state HeatCmdValid
    en:
    VentCmd = TRUE;
  (default) -> HeatCmdInvalid
  HeatCmdInvalid -> HeatCmdValid : /* 指令有效 */
      | [enVentLvlSts.EN_VENT_LVL_OFF != API_VentCmd ...
      | && TRUE == VentCfg && TRUE == VentFlg]
  HeatCmdValid -> HeatCmdInvalid : /* 指令无效 */
      | [enVentLvlSts.EN_VENT_LVL_OFF == API_VentCmd ...
      | || TRUE != VentCfg || TRUE != VentFlg]
  data: API_VentCmd input Enum: enVentLvlSts; VentCfg input uint8; TRUE parameter; VentCmd output uint8; FALSE parameter; VentFlg input uint8

== stateflow chart Appl_VentFault_CtrlModel/LogicCtrl/VentDiagnoseCtrl/VentCommandDeal/VentCmdAquireFunction2/VentCmdAquireFunction ==
  state HeatCmdInvalid
    en:
    VentCmd = FALSE;
  state HeatCmdValid
    en:
    VentCmd = TRUE;
  (default) -> HeatCmdInvalid
  HeatCmdInvalid -> HeatCmdValid : /* 指令有效 */
      | [enVentLvlSts.EN_VENT_LVL_OFF != API_VentCmd ...
      | && TRUE == VentCfg && TRUE == VentFlg]
  HeatCmdValid -> HeatCmdInvalid : /* 指令无效 */
      | [enVentLvlSts.EN_VENT_LVL_OFF == API_VentCmd ...
      | || TRUE != VentCfg || TRUE != VentFlg]
  data: API_VentCmd input Enum: enVentLvlSts; VentCfg input uint8; TRUE parameter; VentCmd output uint8; FALSE parameter; VentFlg input uint8

== stateflow chart Appl_VentFault_CtrlModel/LogicCtrl/VentDiagnoseCtrl/VentDiagnoseDeal/VentCmdDiagnoseFunction1/VentCmdDiagnose ==
  state HeatCmdDiagnosis
    state CmdShortToPower
      ex:
      ShortTimer = 0;
      (default) -> (junction 25)
      CmdShortToPower -> (junction 25) [order 1]
      (junction 25) -> (junction 28) [order 1] : /* 未超时 */
          | [CAL_VentCmdShortTime > ShortTimer]
      (junction 25) -> (junction 30) [order 2] : {/*设置DTC故障标志位，关闭事件报文主驾通风档位*/
          | ShortTimer = CAL_VentCmdShortTime;
          | VentCmdFault = enVentCmdFault.EN_VENT_FAULT_LOAD;
          | VentCmdFault4DTC = enVentCmdFault.EN_VENT_FAULT_LOAD;
          | }
      (junction 28) -> (junction 32) : {ShortTimer++;}
      (junction 32) -> (junction 30)
      (junction 30) -> (junction 35)
    state Default
      en:
      OpenTimer = 0;
      ShortTimer = 0;
      VentCmdFault =  enVentCmdFault.EN_VENT_FAULT_NONE;
      VentCmdFault4DTC =  enVentCmdFault.EN_VENT_FAULT_NONE;
    state CmdOpenLoad
      ex:
      OpenTimer = 0;
      (default) -> (junction 46)
      CmdOpenLoad -> (junction 46) [order 1]
      (junction 46) -> (junction 43) [order 1] : /* 未超时 */
          | [CAL_VentCmdOpenTime > OpenTimer]
      (junction 46) -> (junction 47) [order 2] : {/*设置DTC故障标志位，关闭事件报文主驾通风档位*/
          | OpenTimer = CAL_VentCmdOpenTime;
          | VentCmdFault = enVentCmdFault.EN_VENT_FAULT_OPEN;
          | VentCmdFault4DTC = enVentCmdFault.EN_VENT_FAULT_OPEN;
          | }
      (junction 43) -> (junction 48) : {OpenTimer++;}
      (junction 48) -> (junction 47)
      (junction 47) -> (junction 40)
    (junction 78) -> CmdShortToPower [order 1] : [FaultType ==enVentCmdFault.EN_VENT_FAULT_LOAD]
    Default -> CmdShortToPower [order 1] : /* pwm输出为高 */
        | [TRUE == VentCmdIO]
    CmdShortToPower -> Default [order 1] : /* pwm输出为低 */
        | [FALSE == VentCmdIO]
    (default) -> (junction 78)
    (junction 78) -> Default [order 3]
    (junction 78) -> CmdOpenLoad [order 2] : [FaultType ==enVentCmdFault.EN_VENT_FAULT_OPEN]
    Default -> CmdOpenLoad [order 2] : /* pwm输出为低 且不为 3档*/
        | [FALSE == VentCmdIO ...
        | && VentLvl != enVentLvlSts.EN_VENT_LVL_3]
    CmdOpenLoad -> Default [order 1] : /* pwm输出为高 或为3档*/
        | [TRUE == VentCmdIO ...
        | || VentLvl == enVentLvlSts.EN_VENT_LVL_3]
  state VentCmdClose
    en:
    OpenTimer = 0;
    ShortTimer = 0;
    VentCmdFault = enVentCmdFault.EN_VENT_FAULT_NONE;
    ex:
    VentCmdFault4DTC = FaultType;
  (default) -> VentCmdClose
  VentCmdClose -> HeatCmdDiagnosis : /* 通风CMD */
      | [TRUE == VentCmd]
  HeatCmdDiagnosis -> VentCmdClose : /* 无通风CMD */
      | [TRUE != VentCmd]
  data: VentCmdIO input Enum: enHeatIoSts; VentCmd input uint8; VentCmdFault output Enum: enVentCmdFault; ShortTimer local uint16; OpenTimer local uint16; CAL_VentCmdShortTime parameter; CAL_VentCmdOpenTime parameter; TRUE parameter; FALSE parameter; VentCmdFault4DTC output uint8; FaultType input Enum: enVentCmdFault; VentLvl input Enum: enVentLvlSts

== stateflow chart Appl_VentFault_CtrlModel/LogicCtrl/VentDiagnoseCtrl/VentDiagnoseDeal/VentCmdDiagnoseFunction2/VentCmdDiagnose ==
  state HeatCmdDiagnosis
    state CmdShortToPower
      ex:
      ShortTimer = 0;
      (default) -> (junction 25)
      CmdShortToPower -> (junction 25) [order 1]
      (junction 25) -> (junction 28) [order 1] : /* 未超时 */
          | [CAL_VentCmdShortTime > ShortTimer]
      (junction 25) -> (junction 30) [order 2] : {/*设置DTC故障标志位，关闭事件报文主驾通风档位*/
          | ShortTimer = CAL_VentCmdShortTime;
          | VentCmdFault = enVentCmdFault.EN_VENT_FAULT_LOAD;
          | VentCmdFault4DTC = enVentCmdFault.EN_VENT_FAULT_LOAD;
          | }
      (junction 28) -> (junction 32) : {ShortTimer++;}
      (junction 32) -> (junction 30)
      (junction 30) -> (junction 35)
    state Default
      en:
      OpenTimer = 0;
      ShortTimer = 0;
      VentCmdFault =  enVentCmdFault.EN_VENT_FAULT_NONE;
      VentCmdFault4DTC =  enVentCmdFault.EN_VENT_FAULT_NONE;
    state CmdOpenLoad
      ex:
      OpenTimer = 0;
      (default) -> (junction 46)
      CmdOpenLoad -> (junction 46) [order 1]
      (junction 46) -> (junction 43) [order 1] : /* 未超时 */
          | [CAL_VentCmdOpenTime > OpenTimer]
      (junction 46) -> (junction 47) [order 2] : {/*设置DTC故障标志位，关闭事件报文主驾通风档位*/
          | OpenTimer = CAL_VentCmdOpenTime;
          | VentCmdFault = enVentCmdFault.EN_VENT_FAULT_OPEN;
          | VentCmdFault4DTC = enVentCmdFault.EN_VENT_FAULT_OPEN;
          | }
      (junction 43) -> (junction 48) : {OpenTimer++;}
      (junction 48) -> (junction 47)
      (junction 47) -> (junction 40)
    (junction 78) -> CmdShortToPower [order 1] : [FaultType ==enVentCmdFault.EN_VENT_FAULT_LOAD]
    Default -> CmdShortToPower [order 1] : /* pwm输出为高 */
        | [TRUE == VentCmdIO]
    CmdShortToPower -> Default [order 1] : /* pwm输出为低 */
        | [FALSE == VentCmdIO]
    (default) -> (junction 78)
    (junction 78) -> Default [order 3]
    (junction 78) -> CmdOpenLoad [order 2] : [FaultType ==enVentCmdFault.EN_VENT_FAULT_OPEN]
    Default -> CmdOpenLoad [order 2] : /* pwm输出为低 且不为 3档*/
        | [FALSE == VentCmdIO ...
        | && VentLvl != enVentLvlSts.EN_VENT_LVL_3]
    CmdOpenLoad -> Default [order 1] : /* pwm输出为高 或为3档*/
        | [TRUE == VentCmdIO ...
        | || VentLvl == enVentLvlSts.EN_VENT_LVL_3]
  state VentCmdClose
    en:
    OpenTimer = 0;
    ShortTimer = 0;
    VentCmdFault = enVentCmdFault.EN_VENT_FAULT_NONE;
    ex:
    VentCmdFault4DTC = FaultType;
  (default) -> VentCmdClose
  VentCmdClose -> HeatCmdDiagnosis : /* 通风CMD */
      | [TRUE == VentCmd]
  HeatCmdDiagnosis -> VentCmdClose : /* 无通风CMD */
      | [TRUE != VentCmd]
  data: VentCmdIO input Enum: enHeatIoSts; VentCmd input uint8; VentCmdFault output Enum: enVentCmdFault; ShortTimer local uint16; OpenTimer local uint16; CAL_VentCmdShortTime parameter; CAL_VentCmdOpenTime parameter; TRUE parameter; FALSE parameter; VentCmdFault4DTC output uint8; FaultType input Enum: enVentCmdFault; VentLvl input Enum: enVentLvlSts

== stateflow chart Appl_VentFault_CtrlModel/UpDataInputInfo/InputSignalProcess/PWM_Process/GetFaultType/getFaultType/Chart ==
  (default) -> (junction 1)
  (junction 1) -> (junction 7) [order 2] : [/*PWM短地、开路*/
      | VentPWMGS == TRUE]
  (junction 1) -> (junction 3) [order 1] : [/*PWM短电源*/
      | VentPWMSP == TRUE]
  (junction 7) -> (junction 9) : {VentPWMFault = enVentCmdFault.EN_VENT_FAULT_OPEN}
  (junction 1) -> (junction 11) [order 3] : {VentPWMFault = enVentCmdFault.EN_VENT_FAULT_NONE}
  (junction 3) -> (junction 5) : {VentPWMFault = enVentCmdFault.EN_VENT_FAULT_LOAD}
  (junction 9) -> (junction 11)
  (junction 5) -> (junction 11)
  (junction 11) -> (junction 15)
  data: VentPWMGS input uint8; TRUE parameter; VentPWMFault output uint8; VentPWMSP input uint8

== stateflow chart Appl_VentFault_CtrlModel/UpDataInputInfo/InputSignalProcess/PWM_Process/GetFaultType ==
  state FaultType = getFaultType(ShortGND,ShortPWR) [function]
  state GetFaultType
    du:
    DrFaultType = getFaultType(VentFault_DrPWMShortGND,VentFault_PaPWMShortPWR);
    PaFaultType = getFaultType(VentFault_DrPWMShortPWR,VentFault_3rdPWMShortGND);
    ThirdFaultType = getFaultType(VentFault_PaPWMShortGND,VentFault_3rdPWMShortPWR);
  (default) -> GetFaultType
  data: FaultType function_output; ShortGND function_input; ShortPWR function_input; VentFault_DrPWMShortGND input; VentFault_DrPWMShortPWR input; EN_HEAT_FAULT_GND local double; EN_HEAT_FAULT_NONE local double; EN_HEAT_FAULT_OPEN local double; TRUE local double; VentFault_PaPWMShortGND input; VentFault_PaPWMShortPWR input; VentFault_3rdPWMShortGND input; VentFault_3rdPWMShortPWR input; DrFaultType output Enum: enHeatCmdFault; PaFaultType output Enum: enHeatCmdFault; ThirdFaultType output Enum: enHeatCmdFault
